simulink model "autopilot"  (R2024b)
settings: Solver=FixedStepAuto  StartTime=0.0  StopTime=10.0  FixedStep=5/1000  RelTol=1e-3
settings Model: DataDictionary=example_datadict.sldd  Creator=zhanfuyu  LastModifiedBy=CETCA
settings OptimizationCC: ReuseModelBlockBuffer=off
settings RTWCC: GPUComputeCapability=3.5

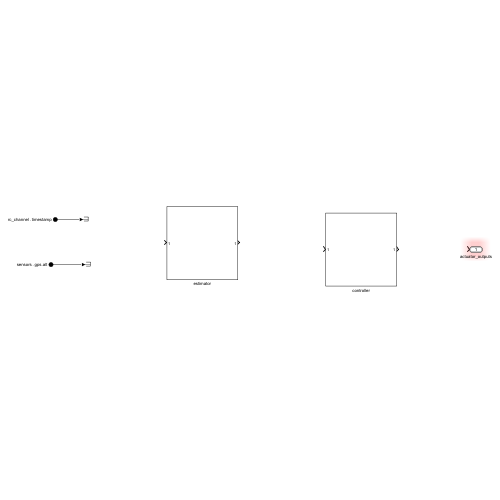
[thumbnail: Simulink's stored preview of the top-level diagram]
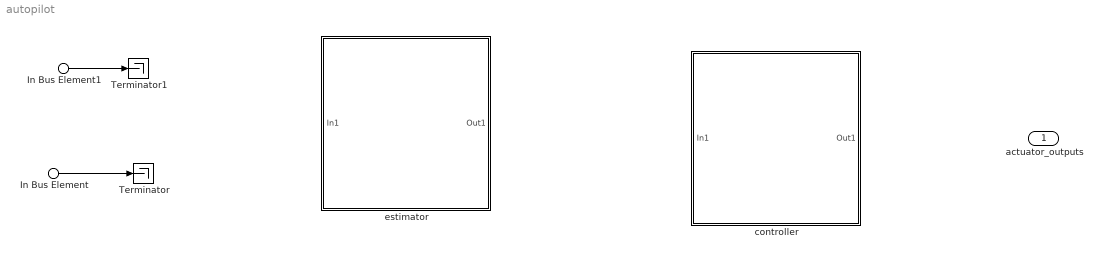
== system autopilot ==
  In Bus Element1 : Inport  PortName=rc_channel  Element=timestamp
  In Bus Element : Inport  Port=2  PortName=sensors  Element=gps.alt
  Terminator : Terminator
  Terminator1 : Terminator
  controller : Subsystem
  estimator : Subsystem
  actuator_outputs : Outport  OutDataTypeStr=Bus: actuator_outputs_s
  wires:
  In Bus Element/1 -> Terminator/1
  In Bus Element1/1 -> Terminator1/1

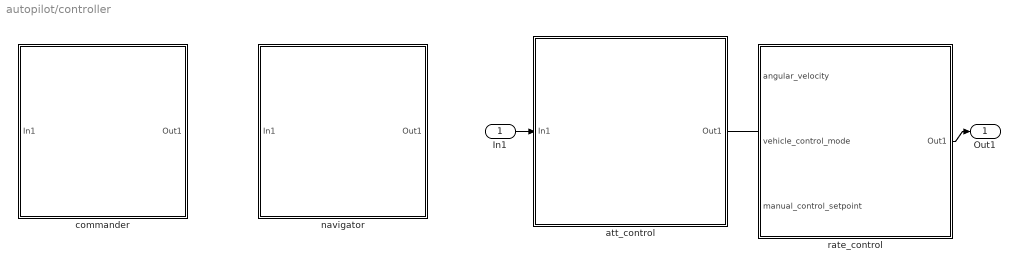
== system autopilot/controller ==
  In1 : Inport
  att_control : Subsystem
  commander : Subsystem
  navigator : Subsystem
  rate_control : Subsystem
  Out1 : Outport
  wires:
  In1/1 -> att_control/1(In1)
  att_control/1(Out1) -> ?
  rate_control/1(Out1) -> Out1/1

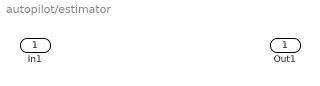
== system autopilot/estimator ==
  In1 : Inport
  Out1 : Outport

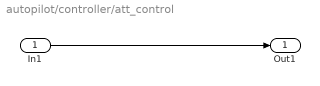
== system autopilot/controller/att_control ==
  In1 : Inport
  Out1 : Outport
  wires:
  In1/1 -> Out1/1

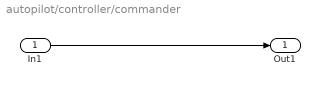
== system autopilot/controller/commander ==
  In1 : Inport
  Out1 : Outport
  wires:
  In1/1 -> Out1/1

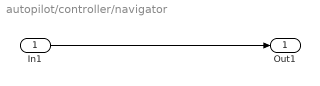
== system autopilot/controller/navigator ==
  In1 : Inport
  Out1 : Outport
  wires:
  In1/1 -> Out1/1

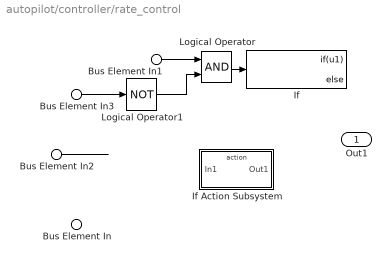
== system autopilot/controller/rate_control ==
  Bus Element In : Inport  PortName=angular_velocity  Element=signal1
  Bus Element In1 : Inport  Port=2  PortName=vehicle_control_mode  Element=flag_control_manual_enabled
  Bus Element In3 : Inport  Port=2  PortName=vehicle_control_mode  Element=flag_control_attitude_enabled
  Bus Element In2 : Inport  Port=3  PortName=manual_control_setpoint
  If : If  IfExpression=u1
  If Action Subsystem : Subsystem  TreatAsAtomicUnit=on
  Logical Operator : Logic  AllPortsSameDT=off  OutDataTypeStr=boolean
  Logical Operator1 : Logic  Operator=NOT  AllPortsSameDT=off  OutDataTypeStr=boolean
  Out1 : Outport
  wires:
  Bus Element In1/1 -> Logical Operator/1
  Bus Element In3/1 -> Logical Operator1/1
  Logical Operator1/1 -> Logical Operator/2
  Logical Operator/1 -> If/1
  Bus Element In2/1 -> ?

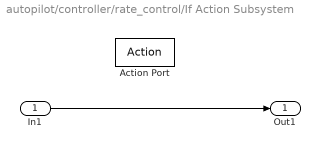
== system autopilot/controller/rate_control/If Action Subsystem ==
  In1 : Inport
  Action Port : ActionPort
  Out1 : Outport
  wires:
  In1/1 -> Out1/1
